simulink model "factory"  (Simulink 8.8)
settings: Solver=ode45  StartTime=0.0  StopTime=30  RelTol=1e-3  EnableMultiTasking=on
PreLoadFcn:
  | Factory
InitFcn:
  | Factory
values from neighbouring files (symbols this model uses):
  JntMax0 = 4.5    [Robot.m]
  JntMin0 = -0.5    [Robot.m]
  PID0 = [0.001 0.002 0.001]    [Controller.m]
  PID1 = [230 75 -0.469]    [Controller.m]
  PID2 = [40 60 -0.5]    [Controller.m]
  Pump0d = [PT0 1]    [Robot.m]
  Pump0n = PK0    [Robot.m]
  Pump0sat = PM0    [Robot.m]
  StartX = 0    [Controller.m]
undefined symbols (not defined in the file or in its folder): Amp1d, Amp1n, Amp2d, Amp2n, AmpSat1, AmpSat2, BackEMF1, BackEMF2, Elec1d, Elec1n, Elec2d, Elec2n, FB0, FB1, FB2, Gear1, Gear2, Grav, InitQ0, InitQ1, InitQ2, JntMax1, JntMax2, JntMin1, JntMin2, L1, L2, Mech0d, Mech0n, Mech1d, Mech1n, Mech2d, Mech2n, TConst1, TConst2
libraries: simulink x9, vrlib x1
settings Model: Creator=Leos  LastModifiedBy=Graham
settings DataIOCC: LimitDataPoints=off
settings OptimizationCC: ExpressionDepthLimit=2147483647
settings DebuggingCC: SolverPrmCheckMsg=warning
settings ConfigComp: CovSFcnEnable=off

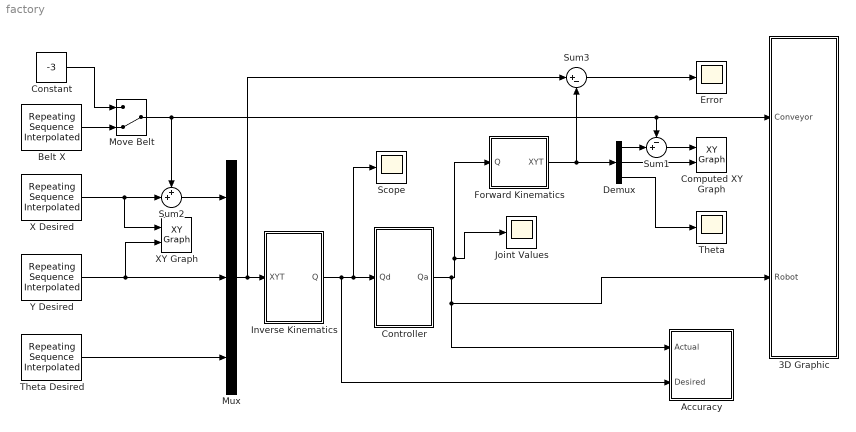
== system factory ==
  3D Graphic : Subsystem
  Accuracy : Subsystem
  Belt X : simulink/Sources/Repeating Sequence Interpolated  OutValues=BeltX  TimeValues=BeltTime  LookUpMeth=Interpolation-Use End Values  tsamp=SampleTime  OutMin=[]  OutMax=[]  OutDataTypeStr=double  OutputDataTypeScalingMode=double  OutDataType=fixdt(0,8)  OutScaling=2^-10
  Computed XY Graph : simulink/Sinks/XY Graph  xmin=-1  xmax=8  ymin=0  ymax=3  st=-1
  Constant : Constant  Value=-3
  Controller : Subsystem
  Demux : Demux  Outputs=3
  Error : Scope
  Forward Kinematics : Subsystem
  Inverse Kinematics : Subsystem
  Joint Values : Scope
  Move Belt : ManualSwitch  CurrentSetting=0
  Mux : Mux  Inputs=3
  Scope : Scope
  Sum1 : Sum  Inputs=-+|
  Sum2 : Sum  Inputs=++|
  Sum3 : Sum  Inputs=|+-
  Theta : Scope
  Theta Desired : simulink/Sources/Repeating Sequence Interpolated  OutValues=Td  TimeValues=Time  LookUpMeth=Interpolation-Use End Values  tsamp=SampleTime  OutMin=[]  OutMax=[]  OutDataTypeStr=double  OutputDataTypeScalingMode=double  OutDataType=fixdt(0,8)  OutScaling=2^-10
  X Desired : simulink/Sources/Repeating Sequence Interpolated  OutValues=Xd  TimeValues=Time  LookUpMeth=Interpolation-Use End Values  tsamp=SampleTime  OutMin=[]  OutMax=[]  OutDataTypeStr=double  OutputDataTypeScalingMode=double  OutDataType=fixdt(0,8)  OutScaling=2^-10
  XY Graph : simulink/Sinks/XY Graph  xmin=-1  xmax=8  ymin=0  ymax=3  st=-1
  Y Desired : simulink/Sources/Repeating Sequence Interpolated  OutValues=Yd  TimeValues=Time  LookUpMeth=Interpolation-Use End Values  tsamp=SampleTime  OutMin=[]  OutMax=[]  OutDataTypeStr=double  OutputDataTypeScalingMode=double  OutDataType=fixdt(0,8)  OutScaling=2^-10
  wires:
  X Desired/1 -> Sum2/2, XY Graph/1
  Y Desired/1 -> Mux/2, XY Graph/2
  Sum2/1 -> Mux/1
  Demux/2 -> Computed XY Graph/2
  Forward Kinematics/1(XYT) -> Sum3/2, Demux/1
  Demux/3 -> Theta/1
  Sum1/1 -> Computed XY Graph/1
  Demux/1 -> Sum1/2
  Sum3/1 -> Error/1
  Constant/1 -> Move Belt/1
  Move Belt/1 -> Sum1/1, 3D Graphic/1(Conveyor), Sum2/1
  Belt X/1 -> Move Belt/2
  Controller/1(Qa) -> 3D Graphic/2(Robot), Accuracy/1(Actual), Joint Values/1, Forward Kinematics/1(Q)
  Inverse Kinematics/1(Q) -> Accuracy/2(Desired), Controller/1(Qd), Scope/1
  Theta Desired/1 -> Mux/3
  Mux/1 -> Sum3/1, Inverse Kinematics/1(XYT)

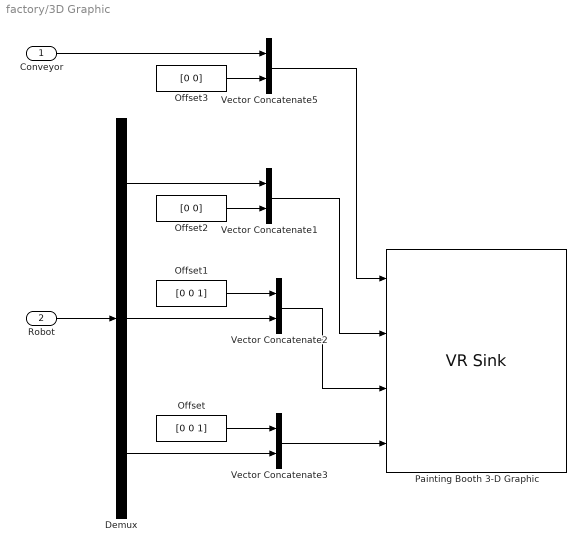
== system factory/3D Graphic ==
  Conveyor : Inport
  Robot : Inport  Port=2
  Demux : Demux  Outputs=3
  Offset : Constant  Value=[0 0 1]
  Offset1 : Constant  Value=[0 0 1]
  Offset2 : Constant  Value=[0 0]
  Offset3 : Constant  Value=[0 0]
  Painting Booth 3-D Graphic : vrlib/VR Sink  InstantiateOnLoad=on  SampleTime=-1  ViewEnable=on  RemoteChange=off  RemoteView=off  FieldsWritten=Truck.translation.3.1.1.double#Q0.translation.3.1.1.double#Q1.rotation.4.1.1.double#Q2.rotation.4.1.1.double  WorldFileName=FACTORY.WRL  AutoView=on  VideoDimensions=[]  AllowVariableSize=off  FigureProperties="{'Position', 'Name', 'Viewpoint', 'CameraBound', 'CameraDirection', 'CameraPosition', 'CameraUpVector', 'ZoomFactor', 'Antialiasing', 'Headlight', 'Lighting', 'NavPanel', 'Sound', 'StatusBar', 'Stereo3D', 'Stereo3DCameraOffset', 'Stereo3DHIT', 'ToolBar', 'Textures', 'Transparency', 'Triad', 'Wireframe', 'NavZones', 'NavMode', 'NavSpeed', 'CaptureFileFormat', 'CaptureFileName', 'Record2DCompressMethod', 'Record2DCompressQuality', 'Record2D', 'Record2DFileName', 'Record2DFPS'; [5.0000000000000000e+00   9.2000000000000000e+01   5.7600000000000000e+02   3.5000000000000000e+02], '', '_untitled_1', 'on', [0.0000000000000000e+00   0.0000000000000000e+00  -1.0000000000000000e+00], [0.0000000000000000e+00   0.0000000000000000e+00   0.0000000000000000e+00], [0.0000000000000000e+00   1.0000000000000000e+00   0.0000000000000000e+00], [1.0000000000000000e+00], 'on', 'off', 'on', 'halfbar', 'on', 'on', 'off', [1.0000000149011612e-01], [0.0000000000000000e+00], 'on', 'on', 'on', 'none', 'off', 'off', 'walk', 'normal', 'tif', '%f_anim_%n.tif', 'auto', [7.5000000000000000e+01], 'off', '%f_anim_%n.avi', 'auto'}"
  Vector Concatenate{1..3,5} (4 alike) : Concatenate
  wires:
  Vector Concatenate5/1 -> Painting Booth 3-D Graphic/1
  Vector Concatenate1/1 -> Painting Booth 3-D Graphic/2
  Vector Concatenate2/1 -> Painting Booth 3-D Graphic/3
  Vector Concatenate3/1 -> Painting Booth 3-D Graphic/4
  Offset/1 -> Vector Concatenate3/1
  Demux/3 -> Vector Concatenate3/2
  Offset1/1 -> Vector Concatenate2/1
  Demux/2 -> Vector Concatenate2/2
  Demux/1 -> Vector Concatenate1/1
  Offset2/1 -> Vector Concatenate1/2
  Offset3/1 -> Vector Concatenate5/2
  Conveyor/1 -> Vector Concatenate5/1
  Robot/1 -> Demux/1

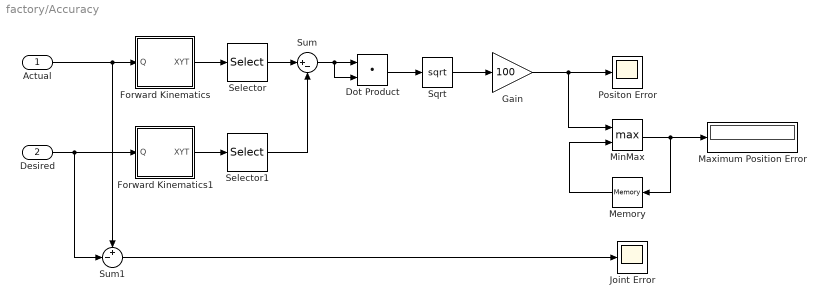
== system factory/Accuracy ==
  Actual : Inport
  Desired : Inport  Port=2
  Dot Product : DotProduct  InputSameDT=on  OutDataTypeStr=Inherit: Inherit via internal rule
  Forward Kinematics : Subsystem
  Forward Kinematics1 : Subsystem
  Gain : Gain  Gain=100
  Joint Error : Scope
  Maximum Position Error : Display
  Memory : Memory
  MinMax : MinMax  Function=max  Inputs=2
  Positon Error : Scope
  Selector : Selector  InputPortWidth=3  IndexOptions=Index vector (dialog)  Indices=[1 2]  OutputSizes=1
  Selector1 : Selector  InputPortWidth=3  IndexOptions=Index vector (dialog)  Indices=[1 2]  OutputSizes=1
  Sqrt : Sqrt  SaturateOnIntegerOverflow=on
  Sum : Sum  Inputs=|+-
  Sum1 : Sum  Inputs=+-|
  wires:
  Forward Kinematics/1(XYT) -> Selector/1
  Actual/1 -> Forward Kinematics/1(Q), Sum1/1
  Selector/1 -> Sum/1
  Selector1/1 -> Sum/2
  Sum/1 -> Dot Product/2, Dot Product/1
  Dot Product/1 -> Sqrt/1
  Forward Kinematics1/1(XYT) -> Selector1/1
  Desired/1 -> Forward Kinematics1/1(Q), Sum1/2
  Sum1/1 -> Joint Error/1
  Memory/1 -> MinMax/2
  MinMax/1 -> Memory/1, Maximum Position Error/1
  Sqrt/1 -> Gain/1
  Gain/1 -> MinMax/1, Positon Error/1

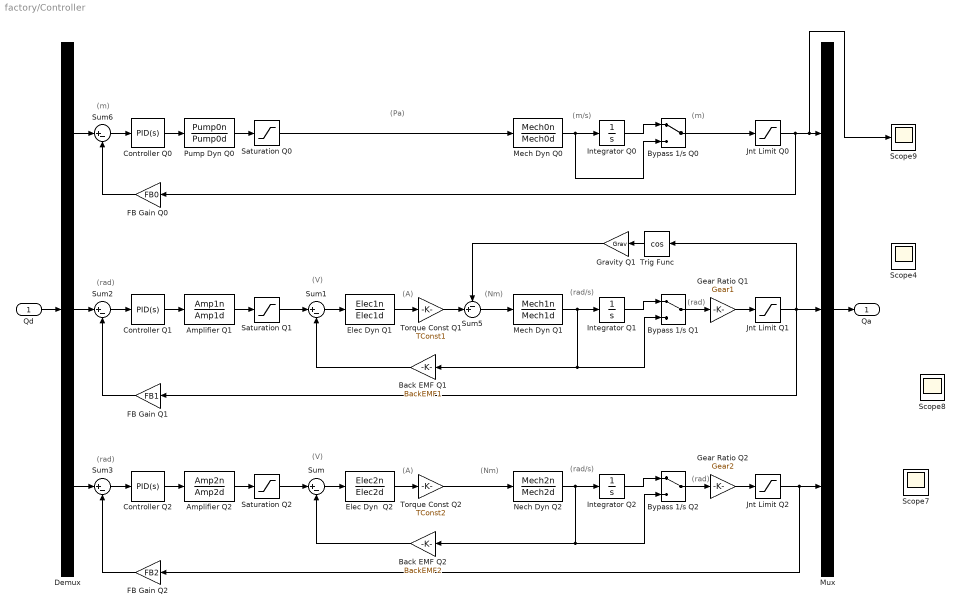
== system factory/Controller ==
  note: (rad)
  note: (V)
  note: (rad/s)
  note: (rad)
  note: (A)
  note: (Nm)
  note: (rad)
  note: (V)
  note: (rad/s)
  note: (rad)
  note: (A)
  note: (Nm)
  note: (m)
  note: (m)
  note: (Pa)
  note: (m/s)
  Qd : Inport
  Amplifier Q1 : TransferFcn  Numerator=Amp1n  Denominator=Amp1d
  Amplifier Q2 : TransferFcn  Numerator=Amp2n  Denominator=Amp2d
  Back EMF Q1 : Gain  Gain=BackEMF1
  Back EMF Q2 : Gain  Gain=BackEMF2
  Bypass 1/s Q0 : ManualSwitch
  Bypass 1/s Q1 : ManualSwitch
  Bypass 1/s Q2 : ManualSwitch
  Controller Q0 : simulink/Continuous/PID Controller  Controller=PID  TimeDomain=Continuous-time  SampleTime=-1  IntegratorMethod=Forward Euler  FilterMethod=Forward Euler  Form=Parallel  UseFilter=on  ControllerParametersSource=internal  P=PID0(1)  I=PID0(2)  D=PID0(3)  N=100  InitialConditionSource=internal  InitialConditionForIntegrator=0  InitialConditionForFilter=0  ExternalReset=none  LimitOutput=off  UpperSaturationLimit=inf  LowerSaturationLimit=-inf  LinearizeAsGain=on  AntiWindupMode=none  Kb=1  TrackingMode=off  Kt=1  PParamMin=[]  PParamMax=[]  IParamMin=[]  IParamMax=[]  DParamMin=[]  DParamMax=[]  NParamMin=[]  NParamMax=[]  KbParamMin=[]  KbParamMax=[]  KtParamMin=[]  KtParamMax=[]  POutMin=[]  POutMax=[]  IOutMin=[]  IOutMax=[]  DOutMin=[]  DOutMax=[]  NOutMin=[]  NOutMax=[]  KbOutMin=[]  KbOutMax=[]  KtOutMin=[]  KtOutMax=[]  IntegratorOutMin=[]  IntegratorOutMax=[]  FilterOutMin=[]  FilterOutMax=[]  SumOutMin=[]  SumOutMax=[]  SumI1OutMin=[]  SumI1OutMax=[]  SumI2OutMin=[]  SumI2OutMax=[]  SumI3OutMin=[]  SumI3OutMax=[]  SumDOutMin=[]  SumDOutMax=[]  SaturationOutMin=[]  SaturationOutMax=[]  IntegratorContinuousStateAttributes=''  IntegratorStateMustResolveToSignalObject=off  IntegratorRTWStateStorageClass=Auto  FilterContinuousStateAttributes=''  FilterStateMustResolveToSignalObject=off  FilterRTWStateStorageClass=Auto  DifferentiatorICPrevScaledInput=0  DifferentiatorOutMin=[]  DifferentiatorOutMax=[]
  Controller Q1 : simulink/Continuous/PID Controller  Controller=PID  TimeDomain=Continuous-time  SampleTime=-1  IntegratorMethod=Forward Euler  FilterMethod=Forward Euler  Form=Parallel  UseFilter=on  ControllerParametersSource=internal  P=PID1(1)  I=PID1(2)  D=PID1(3)  N=100  InitialConditionSource=internal  InitialConditionForIntegrator=0  InitialConditionForFilter=0  ExternalReset=none  LimitOutput=off  UpperSaturationLimit=inf  LowerSaturationLimit=-inf  LinearizeAsGain=on  AntiWindupMode=none  Kb=1  TrackingMode=off  Kt=1  PParamMin=[]  PParamMax=[]  IParamMin=[]  IParamMax=[]  DParamMin=[]  DParamMax=[]  NParamMin=[]  NParamMax=[]  KbParamMin=[]  KbParamMax=[]  KtParamMin=[]  KtParamMax=[]  POutMin=[]  POutMax=[]  IOutMin=[]  IOutMax=[]  DOutMin=[]  DOutMax=[]  NOutMin=[]  NOutMax=[]  KbOutMin=[]  KbOutMax=[]  KtOutMin=[]  KtOutMax=[]  IntegratorOutMin=[]  IntegratorOutMax=[]  FilterOutMin=[]  FilterOutMax=[]  SumOutMin=[]  SumOutMax=[]  SumI1OutMin=[]  SumI1OutMax=[]  SumI2OutMin=[]  SumI2OutMax=[]  SumI3OutMin=[]  SumI3OutMax=[]  SumDOutMin=[]  SumDOutMax=[]  SaturationOutMin=[]  SaturationOutMax=[]  IntegratorContinuousStateAttributes=''  IntegratorStateMustResolveToSignalObject=off  IntegratorRTWStateStorageClass=Auto  FilterContinuousStateAttributes=''  FilterStateMustResolveToSignalObject=off  FilterRTWStateStorageClass=Auto  DifferentiatorICPrevScaledInput=0  DifferentiatorOutMin=[]  DifferentiatorOutMax=[]
  Controller Q2 : simulink/Continuous/PID Controller  Controller=PID  TimeDomain=Continuous-time  SampleTime=-1  IntegratorMethod=Forward Euler  FilterMethod=Forward Euler  Form=Parallel  UseFilter=on  ControllerParametersSource=internal  P=PID2(1)  I=PID2(2)  D=PID2(3)  N=100  InitialConditionSource=internal  InitialConditionForIntegrator=0  InitialConditionForFilter=0  ExternalReset=none  LimitOutput=off  UpperSaturationLimit=inf  LowerSaturationLimit=-inf  LinearizeAsGain=on  AntiWindupMode=none  Kb=1  TrackingMode=off  Kt=1  PParamMin=[]  PParamMax=[]  IParamMin=[]  IParamMax=[]  DParamMin=[]  DParamMax=[]  NParamMin=[]  NParamMax=[]  KbParamMin=[]  KbParamMax=[]  KtParamMin=[]  KtParamMax=[]  POutMin=[]  POutMax=[]  IOutMin=[]  IOutMax=[]  DOutMin=[]  DOutMax=[]  NOutMin=[]  NOutMax=[]  KbOutMin=[]  KbOutMax=[]  KtOutMin=[]  KtOutMax=[]  IntegratorOutMin=[]  IntegratorOutMax=[]  FilterOutMin=[]  FilterOutMax=[]  SumOutMin=[]  SumOutMax=[]  SumI1OutMin=[]  SumI1OutMax=[]  SumI2OutMin=[]  SumI2OutMax=[]  SumI3OutMin=[]  SumI3OutMax=[]  SumDOutMin=[]  SumDOutMax=[]  SaturationOutMin=[]  SaturationOutMax=[]  IntegratorContinuousStateAttributes=''  IntegratorStateMustResolveToSignalObject=off  IntegratorRTWStateStorageClass=Auto  FilterContinuousStateAttributes=''  FilterStateMustResolveToSignalObject=off  FilterRTWStateStorageClass=Auto  DifferentiatorICPrevScaledInput=0  DifferentiatorOutMin=[]  DifferentiatorOutMax=[]
  Demux : Demux  Outputs=3
  Elec Dyn Q1 : TransferFcn  Numerator=Elec1n  Denominator=Elec1d
  Elec Dyn  Q2 : TransferFcn  Numerator=Elec2n  Denominator=Elec2d
  FB Gain Q0 : Gain  Gain=FB0
  FB Gain Q1 : Gain  Gain=FB1
  FB Gain Q2 : Gain  Gain=FB2
  Gear Ratio Q1 : Gain  Gain=Gear1
  Gear Ratio Q2 : Gain  Gain=Gear2
  Gravity Q1 : Gain  Gain=Grav
  Integrator Q0 : Integrator  InitialCondition=InitQ0+StartX
  Integrator Q1 : Integrator  InitialCondition=InitQ1
  Integrator Q2 : Integrator  InitialCondition=InitQ2
  Jnt Limit Q0 : Saturate  UpperLimit=JntMax0  LowerLimit=JntMin0
  Jnt Limit Q1 : Saturate  UpperLimit=JntMax1  LowerLimit=JntMin1
  Jnt Limit Q2 : Saturate  UpperLimit=JntMax2  LowerLimit=JntMin2
  Mech Dyn Q0 : TransferFcn  Numerator=Mech0n  Denominator=Mech0d
  Mech Dyn Q1 : TransferFcn  Numerator=Mech1n  Denominator=Mech1d
  Mux : Mux  Inputs=3
  Nech Dyn Q2 : TransferFcn  Numerator=Mech2n  Denominator=Mech2d
  Pump Dyn Q0 : TransferFcn  Numerator=Pump0n  Denominator=Pump0d
  Saturation Q0 : Saturate  UpperLimit=Pump0sat  LowerLimit=-Pump0sat
  Saturation Q1 : Saturate  UpperLimit=AmpSat1  LowerLimit=-AmpSat1
  Saturation Q2 : Saturate  UpperLimit=AmpSat2  LowerLimit=-AmpSat2
  Scope{4,7..9} (4 alike) : Scope
  Sum{,1..3,6} (5 alike) : Sum  Inputs=|+-
  Sum5 : Sum  Inputs=-+|
  Torque Const Q1 : Gain  Gain=TConst1
  Torque Const Q2 : Gain  Gain=TConst2
  Trig Func : Trigonometry  Operator=cos
  Qa : Outport
  wires:
  Qd/1 -> Demux/1
  Mux/1 -> Qa/1
  Controller Q2/1 -> Amplifier Q2/1
  Sum/1 -> Elec Dyn  Q2/1
  Sum3/1 -> Controller Q2/1
  Elec Dyn  Q2/1 -> Torque Const Q2/1
  Amplifier Q2/1 -> Saturation Q2/1
  Saturation Q2/1 -> Sum/1
  Back EMF Q2/1 -> Sum/2
  Torque Const Q2/1 -> Nech Dyn Q2/1
  FB Gain Q2/1 -> Sum3/2
  Nech Dyn Q2/1 -> Integrator Q2/1, Bypass 1/s Q2/2, Back EMF Q2/1
  Sum1/1 -> Elec Dyn Q1/1
  Elec Dyn Q1/1 -> Torque Const Q1/1
  Amplifier Q1/1 -> Saturation Q1/1
  Saturation Q1/1 -> Sum1/1
  Back EMF Q1/1 -> Sum1/2
  FB Gain Q1/1 -> Sum2/2
  Mech Dyn Q1/1 -> Integrator Q1/1, Bypass 1/s Q1/2, Back EMF Q1/1
  Torque Const Q1/1 -> Sum5/2
  Sum5/1 -> Mech Dyn Q1/1
  Saturation Q0/1 -> Mech Dyn Q0/1
  Sum6/1 -> Controller Q0/1
  Pump Dyn Q0/1 -> Saturation Q0/1
  FB Gain Q0/1 -> Sum6/2
  Trig Func/1 -> Gravity Q1/1
  Gravity Q1/1 -> Sum5/1
  Bypass 1/s Q2/1 -> Gear Ratio Q2/1
  Bypass 1/s Q1/1 -> Gear Ratio Q1/1
  Integrator Q1/1 -> Bypass 1/s Q1/1
  Integrator Q2/1 -> Bypass 1/s Q2/1
  Integrator Q0/1 -> Bypass 1/s Q0/1
  Mech Dyn Q0/1 -> Bypass 1/s Q0/2, Integrator Q0/1
  Jnt Limit Q0/1 -> Scope9/1, Mux/1, FB Gain Q0/1
  Bypass 1/s Q0/1 -> Jnt Limit Q0/1
  Gear Ratio Q1/1 -> Jnt Limit Q1/1
  Jnt Limit Q1/1 -> FB Gain Q1/1, Mux/2, Trig Func/1
  Gear Ratio Q2/1 -> Jnt Limit Q2/1
  Jnt Limit Q2/1 -> FB Gain Q2/1, Mux/3
  Sum2/1 -> Controller Q1/1
  Controller Q1/1 -> Amplifier Q1/1
  Controller Q0/1 -> Pump Dyn Q0/1
  Demux/3 -> Sum3/1
  Demux/1 -> Sum6/1
  Demux/2 -> Sum2/1

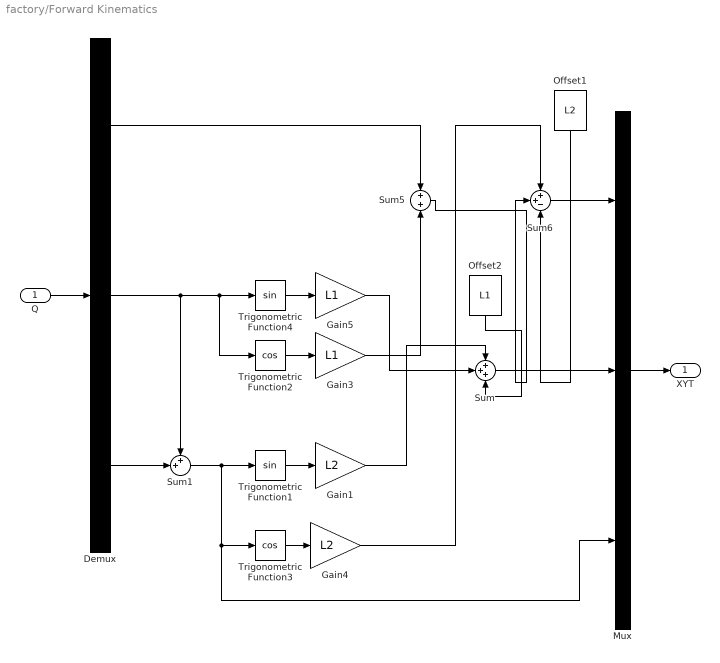
== system factory/Forward Kinematics ==
  Q : Inport
  Demux : Demux  Outputs=3
  Gain1 : Gain  Gain=L2
  Gain3 : Gain  Gain=L1
  Gain4 : Gain  Gain=L2
  Gain5 : Gain  Gain=L1
  Mux : Mux  Inputs=3
  Offset1 : Constant  Value=L2
  Offset2 : Constant  Value=L1
  Sum : Sum  Inputs=+++
  Sum1 : Sum  Inputs=++|
  Sum5 : Sum  Inputs=+|+
  Sum6 : Sum  Inputs=++-
  Trigonometric Function1 : Trigonometry
  Trigonometric Function2 : Trigonometry  Operator=cos
  Trigonometric Function3 : Trigonometry  Operator=cos
  Trigonometric Function4 : Trigonometry
  XYT : Outport
  wires:
  Trigonometric Function1/1 -> Gain1/1
  Trigonometric Function2/1 -> Gain3/1
  Trigonometric Function3/1 -> Gain4/1
  Demux/2 -> Trigonometric Function2/1, Trigonometric Function4/1, Sum1/1
  Trigonometric Function4/1 -> Gain5/1
  Sum/1 -> Mux/2
  Gain1/1 -> Sum/1
  Gain5/1 -> Sum/2
  Demux/3 -> Sum1/2
  Sum1/1 -> Trigonometric Function3/1, Mux/3, Trigonometric Function1/1
  Q/1 -> Demux/1
  Mux/1 -> XYT/1
  Sum6/1 -> Mux/1
  Sum5/1 -> Sum6/2
  Gain4/1 -> Sum6/1
  Gain3/1 -> Sum5/2
  Demux/1 -> Sum5/1
  Offset1/1 -> Sum6/3
  Offset2/1 -> Sum/3

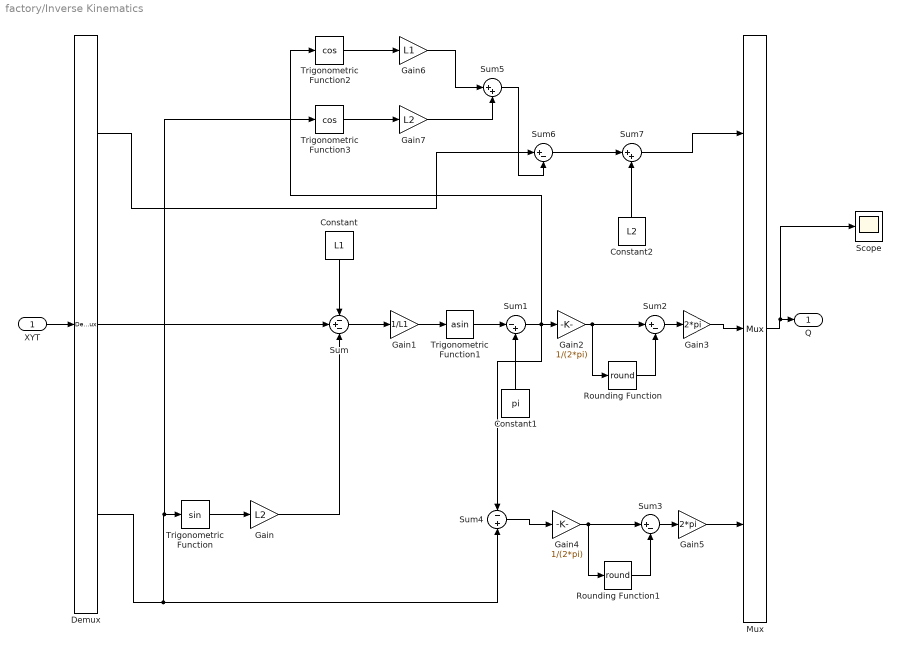
== system factory/Inverse Kinematics ==
  XYT : Inport
  Constant : Constant  Value=L1
  Constant1 : Constant  Value=pi
  Constant2 : Constant  Value=L2
  Demux : Demux  Outputs=3
  Gain : Gain  Gain=L2
  Gain1 : Gain  Gain=1/L1
  Gain2 : Gain  Gain=1/(2*pi)
  Gain3 : Gain  Gain=2*pi
  Gain4 : Gain  Gain=1/(2*pi)
  Gain5 : Gain  Gain=2*pi
  Gain6 : Gain  Gain=L1
  Gain7 : Gain  Gain=L2
  Mux : Mux  Inputs=3
  Rounding Function : Rounding  Operator=round
  Rounding Function1 : Rounding  Operator=round
  Scope : Scope
  Sum : Sum  Inputs=-+-
  Sum1 : Sum  Inputs=|-+
  Sum2 : Sum  Inputs=|+-
  Sum3 : Sum  Inputs=|+-
  Sum4 : Sum  Inputs=-+
  Sum5 : Sum  Inputs=|++
  Sum6 : Sum  Inputs=|+-
  Sum7 : Sum  Inputs=|++
  Trigonometric Function : Trigonometry
  Trigonometric Function1 : Trigonometry  Operator=asin
  Trigonometric Function2 : Trigonometry  Operator=cos
  Trigonometric Function3 : Trigonometry  Operator=cos
  Q : Outport
  wires:
  XYT/1 -> Demux/1
  Mux/1 -> Scope/1, Q/1
  Demux/2 -> Sum/2
  Trigonometric Function/1 -> Gain/1
  Gain/1 -> Sum/3
  Constant/1 -> Sum/1
  Sum/1 -> Gain1/1
  Gain1/1 -> Trigonometric Function1/1
  Sum1/1 -> Sum4/1, Trigonometric Function2/1, Gain2/1
  Constant1/1 -> Sum1/2
  Trigonometric Function1/1 -> Sum1/1
  Gain2/1 -> Sum2/1, Rounding Function/1
  Rounding Function/1 -> Sum2/2
  Sum2/1 -> Gain3/1
  Gain3/1 -> Mux/2
  Gain4/1 -> Sum3/1, Rounding Function1/1
  Rounding Function1/1 -> Sum3/2
  Sum3/1 -> Gain5/1
  Gain5/1 -> Mux/3
  Demux/3 -> Trigonometric Function3/1, Trigonometric Function/1, Sum4/2
  Sum4/1 -> Gain4/1
  Trigonometric Function2/1 -> Gain6/1
  Trigonometric Function3/1 -> Gain7/1
  Gain7/1 -> Sum5/2
  Gain6/1 -> Sum5/1
  Sum5/1 -> Sum6/2
  Demux/1 -> Sum6/1
  Sum6/1 -> Sum7/1
  Constant2/1 -> Sum7/2
  Sum7/1 -> Mux/1

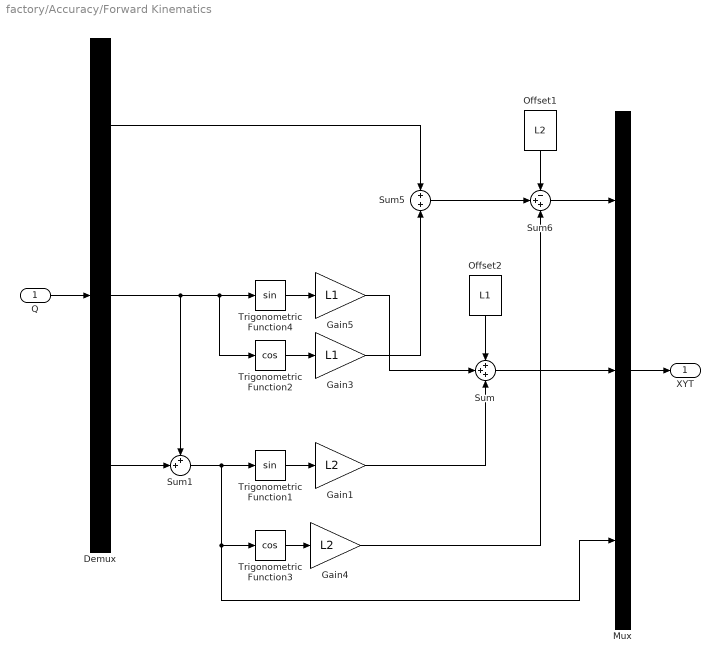
== system factory/Accuracy/Forward Kinematics ==
  Q : Inport
  Demux : Demux  Outputs=3
  Gain1 : Gain  Gain=L2
  Gain3 : Gain  Gain=L1
  Gain4 : Gain  Gain=L2
  Gain5 : Gain  Gain=L1
  Mux : Mux  Inputs=3
  Offset1 : Constant  Value=L2
  Offset2 : Constant  Value=L1
  Sum : Sum  Inputs=+++
  Sum1 : Sum  Inputs=++|
  Sum5 : Sum  Inputs=+|+
  Sum6 : Sum  Inputs=-++
  Trigonometric Function1 : Trigonometry
  Trigonometric Function2 : Trigonometry  Operator=cos
  Trigonometric Function3 : Trigonometry  Operator=cos
  Trigonometric Function4 : Trigonometry
  XYT : Outport
  wires:
  Trigonometric Function1/1 -> Gain1/1
  Trigonometric Function2/1 -> Gain3/1
  Trigonometric Function3/1 -> Gain4/1
  Demux/2 -> Trigonometric Function2/1, Trigonometric Function4/1, Sum1/1
  Trigonometric Function4/1 -> Gain5/1
  Sum/1 -> Mux/2
  Gain1/1 -> Sum/3
  Gain5/1 -> Sum/2
  Offset2/1 -> Sum/1
  Demux/3 -> Sum1/2
  Sum1/1 -> Trigonometric Function3/1, Mux/3, Trigonometric Function1/1
  Q/1 -> Demux/1
  Mux/1 -> XYT/1
  Sum6/1 -> Mux/1
  Sum5/1 -> Sum6/2
  Offset1/1 -> Sum6/1
  Gain4/1 -> Sum6/3
  Gain3/1 -> Sum5/2
  Demux/1 -> Sum5/1

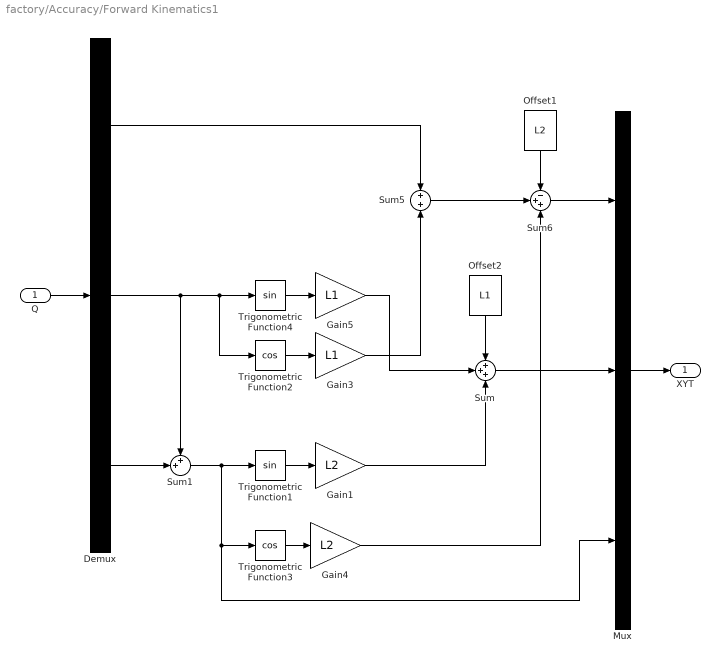
== system factory/Accuracy/Forward Kinematics1 ==
  Q : Inport
  Demux : Demux  Outputs=3
  Gain1 : Gain  Gain=L2
  Gain3 : Gain  Gain=L1
  Gain4 : Gain  Gain=L2
  Gain5 : Gain  Gain=L1
  Mux : Mux  Inputs=3
  Offset1 : Constant  Value=L2
  Offset2 : Constant  Value=L1
  Sum : Sum  Inputs=+++
  Sum1 : Sum  Inputs=++|
  Sum5 : Sum  Inputs=+|+
  Sum6 : Sum  Inputs=-++
  Trigonometric Function1 : Trigonometry
  Trigonometric Function2 : Trigonometry  Operator=cos
  Trigonometric Function3 : Trigonometry  Operator=cos
  Trigonometric Function4 : Trigonometry
  XYT : Outport
  wires:
  Trigonometric Function1/1 -> Gain1/1
  Trigonometric Function2/1 -> Gain3/1
  Trigonometric Function3/1 -> Gain4/1
  Demux/2 -> Trigonometric Function2/1, Trigonometric Function4/1, Sum1/1
  Trigonometric Function4/1 -> Gain5/1
  Sum/1 -> Mux/2
  Gain1/1 -> Sum/3
  Gain5/1 -> Sum/2
  Offset2/1 -> Sum/1
  Demux/3 -> Sum1/2
  Sum1/1 -> Trigonometric Function3/1, Mux/3, Trigonometric Function1/1
  Q/1 -> Demux/1
  Mux/1 -> XYT/1
  Sum6/1 -> Mux/1
  Sum5/1 -> Sum6/2
  Offset1/1 -> Sum6/1
  Gain4/1 -> Sum6/3
  Gain3/1 -> Sum5/2
  Demux/1 -> Sum5/1
